simulink model "relay_feedback_method"  (R2023a)
settings: Solver=VariableStepAuto  StartTime=0.0  StopTime=400  RelTol=1e-3
undefined symbols (not defined in the file or in its folder): simP
settings Model: Creator=pascalbock  LastModifiedBy=pascalbock

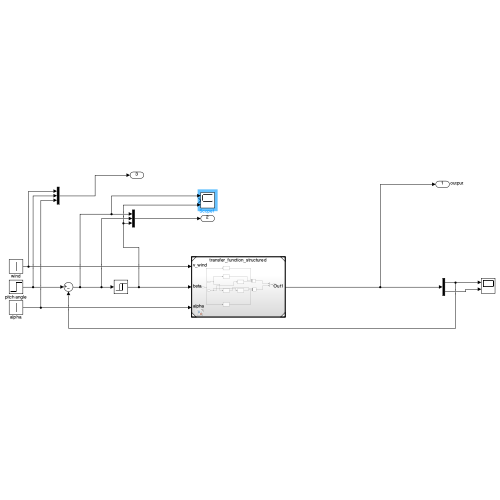
[thumbnail: Simulink's stored preview of the top-level diagram]
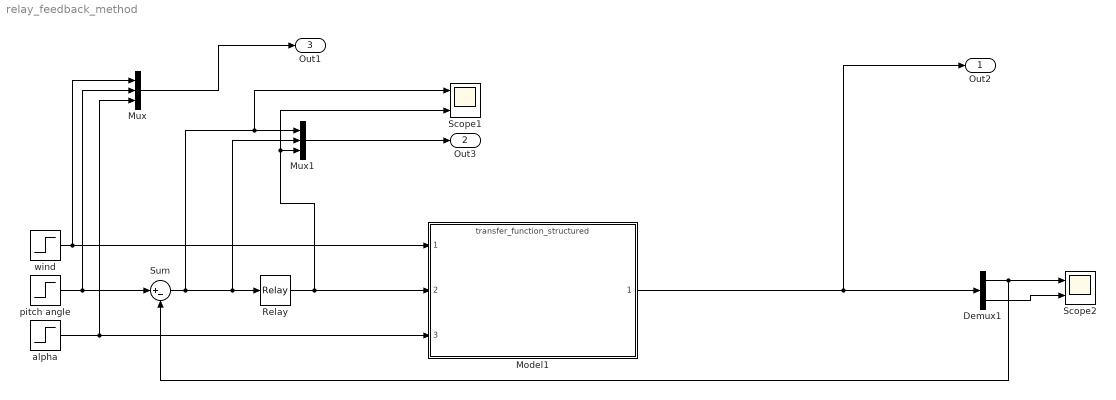
== system relay_feedback_method ==
  Demux1 : Demux  Outputs=2
  Model1 : ModelReference  ModelNameDialog=transfer_function_structured.slx  SimulationMode=Normal  ModelReferenceVersion=1.2
  Mux : Mux  Inputs=3
  Mux1 : Mux  Inputs=3
  Relay : Relay  OnSwitchValue=1  OffSwitchValue=-1  OnOutputValue=-1  OffOutputValue=1
  Scope1 : Scope  NumInputPorts=3
  Scope2 : Scope  NumInputPorts=2
  Sum : Sum  Inputs=|+-
  alpha : Step  Time=simP.step_time  After=0  SampleTime=0
  pitch angle : Step  Time=simP.step_time  After=0  SampleTime=0
  wind : Step  Time=simP.step_time  After=0  SampleTime=0
  Out2 : Outport  SignalName=output
  Out3 : Outport  Port=2
  Out1 : Outport  Port=3
  wires:
  Model1/1 -> Demux1/1, Out2/1
  Demux1/2 -> Scope2/2
  Demux1/1 -> Sum/2, Scope2/1
  Sum/1 -> Mux1/2, Relay/1, Scope1/1, Mux1/1
  wind/1 -> Mux/1, Model1/1
  alpha/1 -> Mux/3, Model1/3
  Mux/1 -> Out1/1
  Mux1/1 -> Out3/1
  pitch angle/1 -> Mux/2, Sum/1
  Relay/1 -> Model1/2, Scope1/3, Mux1/3
